simulink model "Bitwise_AND"  (R2013b)
settings: Solver=ode45  StartTime=0.0  StopTime=10.0  RelTol=1e-3
libraries: translib x1
settings Model: Creator=daltdoer  LastModifiedBy=daltdoer

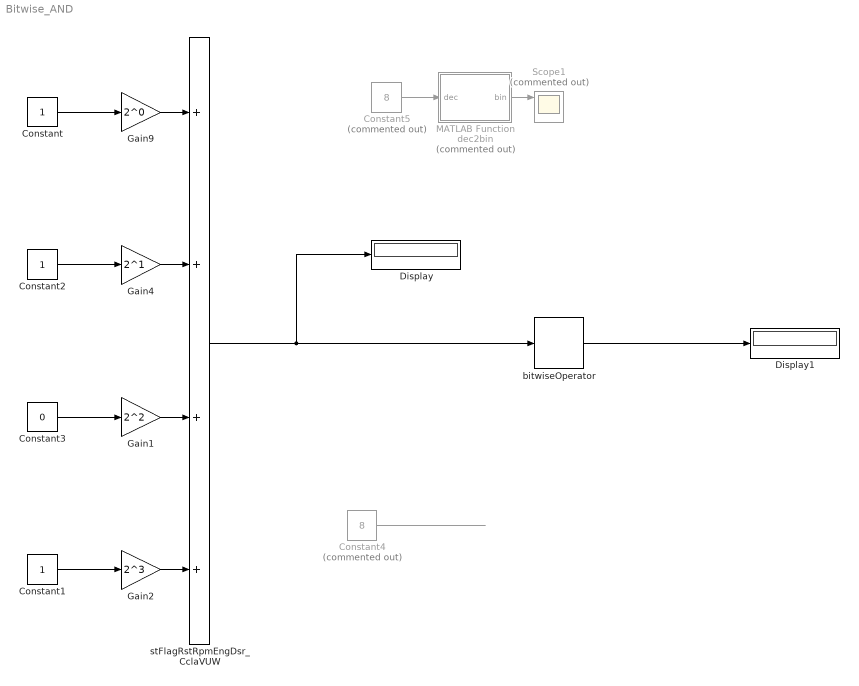
== system Bitwise_AND ==
  Constant : Constant
  Constant1 : Constant
  Constant2 : Constant
  Constant3 : Constant  Value=0
  Constant4 : Constant  Commented=on  Value=8
  Constant5 : Constant  Commented=on  Value=8
  Display : Display
  Display1 : Display
  Gain1 : Gain  Description=#user:sbeukel#  Gain=2^2  OutDataTypeStr=double  mask(TL_Gain){data={'logdata',{'plotchannels',[]},'output',{'type','UInt16','scaling','sc_bin/NonDims/NonDim_bp0'},'gain',{'type','CONTINUOUS'},'autoscaling',{'mode',2},'date',736211.52538202552}}
      settings: CopyFcn=if exist('tl_reset_reviewflag','file')==2,tl_reset_reviewflag(gcbh);end  DeleteFcn=if exist('delete_tlblock','file')==2,delete_tlblock(gcbh);end  NameChangeFcn=if exist('rename_tlblock','file')==2,rename_tlblock(gcbh);end  OpenFcn=if exist('tl_open_blockdlg','file')==2,tl_open_blockdlg(gcbh);else,open_system(gcbh,'parameter');end
      mask Help: eval(['if exist(''tl_online_help'',''file'') == 2, tl_online_help(''Topic'',''TL_Gain''),else, web([''jar:file:///'',matlabroot,''/help/toolbox/simulink/help.jar!/slref/' lower(get_param(gcbh,'Blocktype')) '.html''], ''-helpbrowser''),end'])
      mask Display: plot([0, .9, 0],[.05, .5, .95])
  Gain2 : Gain  Description=#user:sbeukel#  Gain=2^3  OutDataTypeStr=double  mask(TL_Gain){data={'logdata',{'plotchannels',[]},'output',{'type','UInt16','scaling','sc_bin/NonDims/NonDim_bp0'},'gain',{'type','CONTINUOUS'},'autoscaling',{'mode',2},'date',736211.52537923609}}
      settings: CopyFcn=if exist('tl_reset_reviewflag','file')==2,tl_reset_reviewflag(gcbh);end  DeleteFcn=if exist('delete_tlblock','file')==2,delete_tlblock(gcbh);end  NameChangeFcn=if exist('rename_tlblock','file')==2,rename_tlblock(gcbh);end  OpenFcn=if exist('tl_open_blockdlg','file')==2,tl_open_blockdlg(gcbh);else,open_system(gcbh,'parameter');end
      mask Help: eval(['if exist(''tl_online_help'',''file'') == 2, tl_online_help(''Topic'',''TL_Gain''),else, web([''jar:file:///'',matlabroot,''/help/toolbox/simulink/help.jar!/slref/' lower(get_param(gcbh,'Blocktype')) '.html''], ''-helpbrowser''),end'])
      mask Display: plot([0, .9, 0],[.05, .5, .95])
  Gain4 : Gain  Description=#user:sbeukel#  Gain=2^1  OutDataTypeStr=double  mask(TL_Gain){data={'logdata',{'plotchannels',[]},'output',{'type','UInt16','scaling','sc_bin/NonDims/NonDim_bp0'},'gain',{'type','CONTINUOUS'},'autoscaling',{'mode',2},'date',736211.52537853015}}
      settings: CopyFcn=if exist('tl_reset_reviewflag','file')==2,tl_reset_reviewflag(gcbh);end  DeleteFcn=if exist('delete_tlblock','file')==2,delete_tlblock(gcbh);end  NameChangeFcn=if exist('rename_tlblock','file')==2,rename_tlblock(gcbh);end  OpenFcn=if exist('tl_open_blockdlg','file')==2,tl_open_blockdlg(gcbh);else,open_system(gcbh,'parameter');end
      mask Help: eval(['if exist(''tl_online_help'',''file'') == 2, tl_online_help(''Topic'',''TL_Gain''),else, web([''jar:file:///'',matlabroot,''/help/toolbox/simulink/help.jar!/slref/' lower(get_param(gcbh,'Blocktype')) '.html''], ''-helpbrowser''),end'])
      mask Display: plot([0, .9, 0],[.05, .5, .95])
  Gain9 : Gain  Description=#user:sbeukel#  Gain=2^0  OutDataTypeStr=double  mask(TL_Gain){data={'logdata',{'plotchannels',[]},'output',{'type','UInt16','scaling','sc_bin/NonDims/NonDim_bp0'},'gain',{'type','CONTINUOUS'},'autoscaling',{'mode',2},'date',736211.5253767824}}
      settings: CopyFcn=if exist('tl_reset_reviewflag','file')==2,tl_reset_reviewflag(gcbh);end  DeleteFcn=if exist('delete_tlblock','file')==2,delete_tlblock(gcbh);end  NameChangeFcn=if exist('rename_tlblock','file')==2,rename_tlblock(gcbh);end  OpenFcn=if exist('tl_open_blockdlg','file')==2,tl_open_blockdlg(gcbh);else,open_system(gcbh,'parameter');end
      mask Help: eval(['if exist(''tl_online_help'',''file'') == 2, tl_online_help(''Topic'',''TL_Gain''),else, web([''jar:file:///'',matlabroot,''/help/toolbox/simulink/help.jar!/slref/' lower(get_param(gcbh,'Blocktype')) '.html''], ''-helpbrowser''),end'])
      mask Display: plot([0, .9, 0],[.05, .5, .95])
  MATLAB Function dec2bin : MATLAB Function  Commented=on  TreatAsAtomicUnit=on
  Scope1 : Scope  Commented=on  NumInputPorts=3
      settings: YMin=-5~-5~-5  YMax=5~5~5
  bitwiseOperator : translib/Logical/bitwiseOperator  dataType=T_U8  logicop=AND  UseBitMask=on  NumInputPorts=2  BitMask=bin2dec('1011')  BitMaskRealWorld=Stored Integer
      settings: AttributesFormatString=%<dataType>
  stFlagRstRpmEngDsr_CclaVUW : Sum  Description=#user:hobruec#  Inputs=++++  OutDataTypeStr=double  mask(TL_Sum){data={'logdata',{'plotchannels',[]},'output',{'variable','Lc/Scla/Scla_LVAR/stFlagRstRpmEngDsr_SclaVUW'},'autoscaling',{'mode',2},'date',736847.62360315968}}
      settings: CopyFcn=if exist('tl_reset_reviewflag','file')==2,tl_reset_reviewflag(gcbh);end  DeleteFcn=if exist('delete_tlblock','file')==2,delete_tlblock(gcbh);end  NameChangeFcn=if exist('rename_tlblock','file')==2,rename_tlblock(gcbh);end  OpenFcn=if exist('tl_open_blockdlg','file')==2,tl_open_blockdlg(gcbh);else,open_system(gcbh,'parameter');end
      mask Help: eval(['if exist(''tl_online_help'',''file'') == 2, tl_online_help(''Topic'',''TL_Sum''),else, web([''jar:file:///'',matlabroot,''/help/toolbox/simulink/help.jar!/slref/' lower(get_param(gcbh,'Blocktype')) '.html''], ''-helpbrowser''),end'])
      mask Display: plot([-0.05, 1.05, NaN, -0.05, 1.05],[.01, .01, NaN, .99, .99])
  wires:
  Gain9/1 -> stFlagRstRpmEngDsr_CclaVUW/1
  Gain2/1 -> stFlagRstRpmEngDsr_CclaVUW/4
  Gain1/1 -> stFlagRstRpmEngDsr_CclaVUW/3
  Gain4/1 -> stFlagRstRpmEngDsr_CclaVUW/2
  Constant/1 -> Gain9/1
  Constant1/1 -> Gain2/1
  Constant2/1 -> Gain4/1
  Constant3/1 -> Gain1/1
  Constant4/1 -> ?
  stFlagRstRpmEngDsr_CclaVUW/1 -> bitwiseOperator/1, Display/1
  Constant5/1 -> MATLAB Function dec2bin/1(dec)
  MATLAB Function dec2bin/1(bin) -> Scope1/1
  bitwiseOperator/1 -> Display1/1

== matlab function Bitwise_AND/MATLAB Function dec2bin ==
  data: dec input; bin output
function bin = dec_2_bin(dec)

%% Code zur Erzeugung eines Binärcodes aus Dezimalzahl
 
n=0;

j=1; % Erster Eintrag Vektor
n2=zeros(1,30);
n2(j)=2^n; %Zweierpotenz 1. Eintrag 2^0; 2. Eintrag 2^1 usw.

%% Suche wieviel Potenzen man braucht
    
for j=1:30 % zu suchende Zahl bis unendlich möglich 
    
    n2(j)=2^n;
    n=n+1; % Iterative erhöhung der Potenz bis n2(j) >= dec

    if n2(j) >= dec && mod(n2(j),dec)==0 % Wenn Zahl genau der Potenz entspricht 
    
        break;  % Bricht for schleife ab 
        
    elseif n2(j) >= dec && mod(n2(j),dec)~=0  % Wenn Zahl kleiner als höchste Potenz entspricht 
        
        n=n-1;
        break;  % Bricht for schleife ab   
        
    end
end

% n_notw=n        % Ergebnis: Anzahl der Potenzen, die max gebraucht werden
% dec_notw=n2(n)  % Ergebnis in Dezimal

%% Dec in Binär umwandeln 
bin_vec=zeros(1,n);      % Erzeugt Nullvektor
rest_prev=dec;        % Jeweils verbleibender Restwert an Zahlen vor Umrechnung in Binär


for k=1:n

    k_n2_back=n+1-k; % Vektor n2 Zugriff rückwärts
    
    [bin_curr_bit,rest_curr] = current_bin_bit(n2,k,k_n2_back,rest_prev);

     bin_vec(k) = bin_curr_bit(k); % Setzt das aktuelle Bits auf entsprechende Stelle 
     rest_prev = rest_curr;
     
end

% bin_vec = bin_vec % Test

%% Transformation Vektor zu einzelner DezimalZahl
   
bin=0;

for i=1:1:(size(bin_vec,2)) 
    k_n2_back=n+1-i;
    
   bin = bin+bin_vec(k_n2_back)*10^(i-1);
    
end


end

function [bin_curr_bit1,rest_curr1] = current_bin_bit(n2,k,k_n2_back1,rest_prev1)

% Ausgang:
% bin_curr_bit -> Aktuelles Bit 0 oder 1
% rest_curr aktueller Rest für nächstes Bit 

% Eingänge:
% n2 Vektor mit allen Potenzzahl
% k ist aktuelle Postion des Binärvektors von links
% k_n2_back ist aktuelle Postion des Potenzvektors von rechts
% rest_prev -> Restzahl die aufgespalten werden muss
bin_curr_bit1=0;

    if (rest_prev1/n2(k_n2_back1)) < 1 % Wenn sich der Rest nicht durch aktuelle Potenzzahlteilen lässt

        bin_curr_bit1(k) = 0; %wird bit auf 0 gesetzt

        rest_curr1=rest_prev1; % und rest bleibt gleich

    elseif (rest_prev1/n2(k_n2_back1)) >= 1 % Wenn sich der Rest durch aktuelle Potenzzahlteilen lässt

        bin_curr_bit1(k) = 1; % wird aktuelles bit auf 1 gesetzt

        rest_curr1 = mod(rest_prev1,n2(k_n2_back1)); 


    end 
end
